simulink model "ENGN3223_system 1"  (R2025b)
settings: Solver=VariableStepAuto  StartTime=0.0  StopTime=10.0  RelTol=1e-3
values from neighbouring files (symbols this model uses):
  A = [-2.02     1       0 ... (first row only)    [ENGN3223_code 1.m]    (also in ENGN3223_final.m = [X_u              X_w            0              -g; ENGN3223_updated.m = [X_u              X_w            0              -g)
  B = [0.16 ... (first row only)    [ENGN3223_code 1.m]    (also in ENGN3223_final.m = -[X_del               X_del_T; ENGN3223_updated.m = -[X_del               X_del_T)
  K = acker(A,B,desired_poles)    [ENGN3223_code 1.m]    (also in ENGN3223_final.m = place(A,B,desired_poles); ENGN3223_updated.m = place(A,B,desired_poles))

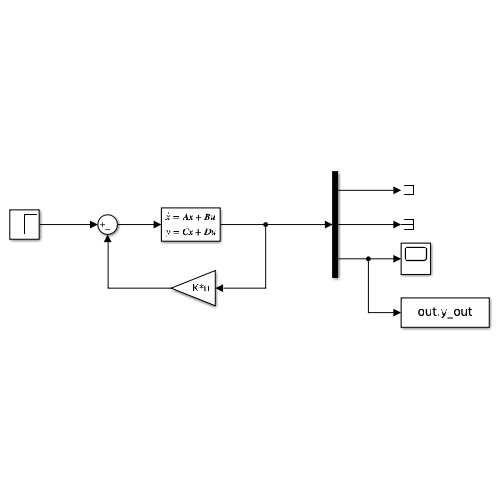
[thumbnail: Simulink's stored preview of the top-level diagram]
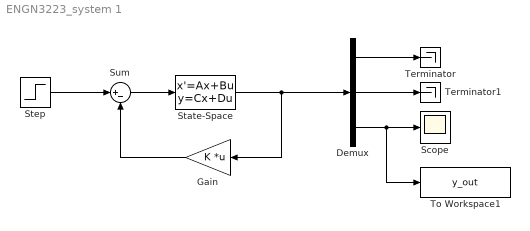
== system ENGN3223_system 1 ==
  Demux : Demux  Outputs=3
  Gain : Gain  Gain=K  Multiplication=Matrix(K*u)
  Scope : Scope
      settings: ActiveDisplayYMinimum=-0.074928366668926577  ActiveDisplayYMaximum=0.67435530002033928
  State-Space : StateSpace  A=A  B=B  C=eye(3)  D=[0;0;0]  InitialCondition=0  ContinuousStateAttributes={'Angle_of_attack','Pitch_rate','Pitch_angle'}
  Step : Step  Time=0  After=0.2  SampleTime=0
  Sum : Sum  Inputs=|+-
  Terminator : Terminator
  Terminator1 : Terminator
  To Workspace1 : ToWorkspace  VariableName=y_out  SaveFormat=Timeseries  SampleTime=-1
  wires:
  Step/1 -> Sum/1
  State-Space/1 -> Demux/1, Gain/1
  Sum/1 -> State-Space/1
  Gain/1 -> Sum/2
  Demux/3 -> To Workspace1/1, Scope/1
  Demux/2 -> Terminator1/1
  Demux/1 -> Terminator/1
